simulink model "ROS_DJI_waypoint_follower"  (R2020b)
settings: Solver=FixedStepDiscrete  StartTime=0.0  StopTime=inf  FixedStep=0.001  RelTol=1e-3  EnableMultiTasking=on
model workspace (MAT data in the model file):
  SL_ROS_VariableLengthArrays_MaxSizes.CommonInfo.ArrayTruncateAction = 'EmitWarning'
  SL_ROS_VariableLengthArrays_MaxSizes.MsgTypeMap = containers.Map
  SL_ROS_VariableLengthArrays_MaxSizes.MsgTypeMap.serialization.keys = {'geometry_msgs/PoseArray', 'sensor_msgs/Joy'}
  SL_ROS_VariableLengthArrays_MaxSizes.MsgTypeMap.serialization.values{1}.PropertyName = 'Poses'
  SL_ROS_VariableLengthArrays_MaxSizes.MsgTypeMap.serialization.values{1}.DataType = 'geometry_msgs/Pose'
  SL_ROS_VariableLengthArrays_MaxSizes.MsgTypeMap.serialization.values{1}.MaxLength = 255
  SL_ROS_VariableLengthArrays_MaxSizes.MsgTypeMap.serialization.values{2}(1).PropertyName = 'Axes'
  SL_ROS_VariableLengthArrays_MaxSizes.MsgTypeMap.serialization.values{2}(1).DataType = 'single'
  SL_ROS_VariableLengthArrays_MaxSizes.MsgTypeMap.serialization.values{2}(1).MaxLength = 4
  SL_ROS_VariableLengthArrays_MaxSizes.MsgTypeMap.serialization.values{2}(2).PropertyName = 'Buttons'
  SL_ROS_VariableLengthArrays_MaxSizes.MsgTypeMap.serialization.values{2}(2).DataType = 'int32'
  SL_ROS_VariableLengthArrays_MaxSizes.MsgTypeMap.serialization.values{2}(2).MaxLength = 128
  SL_ROS_VariableLengthArrays_MaxSizes.MsgTypeMap.serialization.uniformity = 0
  SL_ROS_VariableLengthArrays_MaxSizes.MsgTypeMap.serialization.keyType = 'char'
  SL_ROS_VariableLengthArrays_MaxSizes.MsgTypeMap.serialization.valueType = 'any'
undefined symbols (not defined in the file or in its folder): DJIServiceDroneTaskControl
libraries: robotlib x13, simulink x5, uavutilslib x1, uavalgslib x1
settings Model: EnablePacing=on  Creator=The MathWorks, Inc.  LastModifiedBy=kritika
settings DataIOCC: LimitDataPoints=on  SaveFormat=Array  ReturnWorkspaceOutputs=off
settings OptimizationCC: ZeroExternalMemoryAtStartup=off  ZeroInternalMemoryAtStartup=off  LifeSpan=1  MaxStackSize=64  EfficientTunableParamExpr=on
settings DebuggingCC: SolverPrmCheckMsg=warning  SFUnexpectedBacktrackingDiag=warning  SFNoUnconditionalDefaultTransitionDiag=warning  SFExecutionAtInitializationDiag=none  ArithmeticOperatorsInVariantConditions=warning
settings HardwareCC: ProdBitPerPointer=32  ProdBitPerSizeT=32  ProdBitPerPtrDiffT=32  ProdLargestAtomicFloat=None  ProdIntDivRoundTo=Undefined  ProdEndianess=Unspecified  ProdWordSize=32  ProdHWDeviceType=Generic->Unspecified (assume 32-bit Generic)  TargetHWDeviceType=Generic->Unspecified (assume 32-bit Generic)
settings ModelReferenceCC: PropagateSignalLabelsOutOfModel=off
settings SFSimCC: SimUseLocalCustomCode=off  CustomCodeUndefinedFunction=UseInterfaceOnly  SimTargetLang=C++
settings RTWCC: Description=Embedded Coder  SystemTargetFile=ert.tlc  HardwareBoard=Robot Operating System (ROS)  TLCOptions=-aInlineSetEventsForThisBaseRateFcn=TLC_FALSE -aSuppressMultiTaskScheduler=TLC_FALSE -aRateBasedStepFcn=0  TemplateMakefile=ert_default_tmf  RTWUseLocalCustomCode=off  Toolchain=Catkin  TargetLang=C++
settings CodeAppCC: StateflowObjectComments=on
settings ERTTargetCC: MultiwordLength=2048  ERTCustomFileBanners=off  CodeInterfacePackaging=C++ class  SupportContinuousTime=on  SupportNonInlinedSFcns=on  RemoveResetFunc=off  SupportVariableSizeSignals=on  ModelStepFunctionPrototypeControlCompliant=off  RootIOFormat=Structure reference  ConvertIfToSwitch=off  SuppressUnreachableDefaultCases=off
settings ConfigComp: CovMetricSettings=dw  CovSaveCumulativeToWorkspaceVar=on  CovSaveSingleToWorkspaceVar=on  CovExternalEMLEnable=off  CovSFcnEnable=off

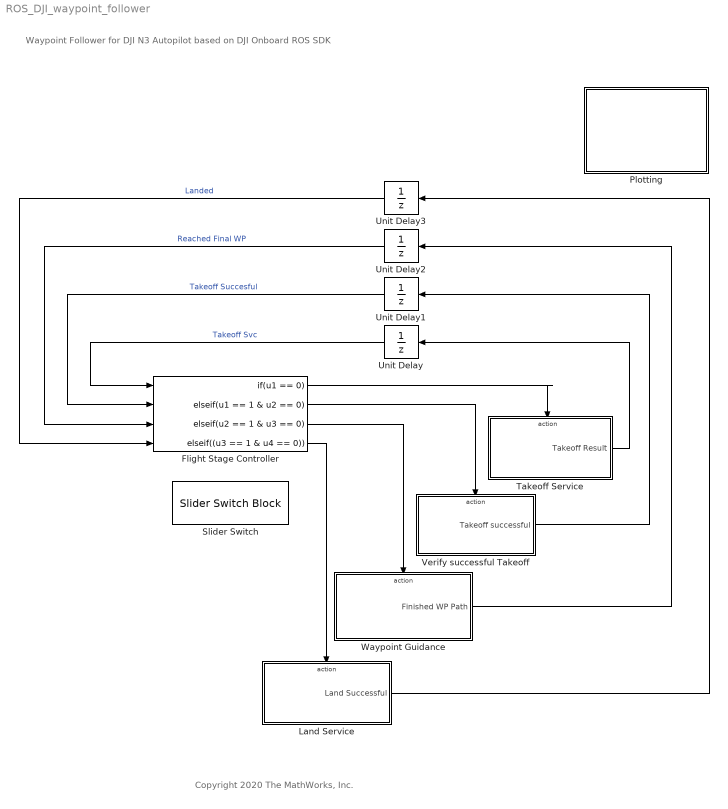
== system ROS_DJI_waypoint_follower ==
  note: Copyright 2020 The MathWorks, Inc.
  note: Waypoint Follower for DJI N3 Autopilot based on DJI Onboard ROS SDK
  Flight Stage Controller : If  NumInputs=4  IfExpression=u1 == 0  ElseIfExpressions=u1 == 1 & u2 == 0, u2 == 1 & u3 == 0, (u3 == 1 & u4 == 0)  ShowElse=off
  Land Service : Subsystem  TreatAsAtomicUnit=on
  Plotting : Subsystem
  Slider Switch : SliderSwitchBlock
      settings: Values={{'Off', 'On'}, [0 1]}
  Takeoff Service : Subsystem
  Unit Delay{,1..3} (4 alike) : UnitDelay  SampleTime=-1  HasFrameUpgradeWarning=on
  Verify successful Takeoff : Subsystem
  Waypoint Guidance : Subsystem
  wires:
  Unit Delay/1 -> Flight Stage Controller/1  "Takeoff Svc"
  Flight Stage Controller/1 -> Takeoff Service/Action
  Takeoff Service/1(Takeoff Result) -> Unit Delay/1
  Flight Stage Controller/2 -> Verify successful Takeoff/Action
  Verify successful Takeoff/1(Takeoff successful) -> Unit Delay1/1
  Unit Delay1/1 -> Flight Stage Controller/2  "Takeoff Succesful"
  Flight Stage Controller/3 -> Waypoint Guidance/Action
  Waypoint Guidance/1(Finished WP Path) -> Unit Delay2/1
  Unit Delay2/1 -> Flight Stage Controller/3  "Reached Final WP"
  Flight Stage Controller/4 -> Land Service/Action
  Land Service/1(Land Successful) -> Unit Delay3/1
  Unit Delay3/1 -> Flight Stage Controller/4  "Landed"

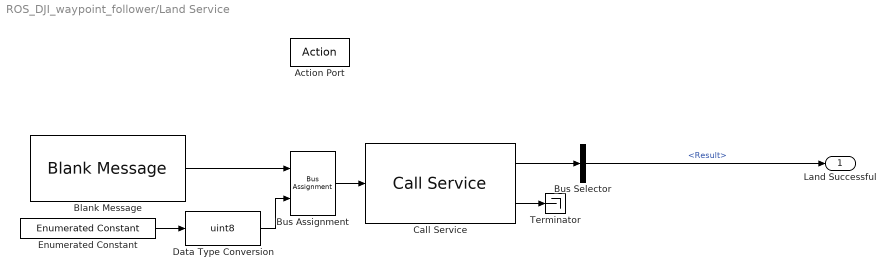
== system ROS_DJI_waypoint_follower/Land Service ==
  Action Port : ActionPort  ActionPortLabel=elseif( (u3 == 1 & u4 == 0))
  Blank Message : robotlib/Blank Message  messageClass=Service Request  entityType=std_srvs/Empty  messageType=std_srvs/EmptyRequest  SampleTime=-1  legacyBusStruct=off
  Bus Assignment : BusAssignment  AssignedSignals=Task
  Bus Selector : BusSelector  OutputSignals=Result
  Call Service : robotlib/Call Service  topicSource=Select from ROS network  service=/dji_sdk/drone_task_control  serviceType=dji_sdk/DroneTaskControl  connectionTimeout=5  keepPersistent=off  ShowErrorCodeOutput=on  legacyBusStruct=off
      settings: SourceProductBaseCode=RR
  Data Type Conversion : DataTypeConversion  OutDataTypeStr=uint8
  Enumerated Constant : simulink/Sources/Enumerated Constant  OutDataTypeStr=Enum: DJIServiceDroneTaskControl  Value=DJIServiceDroneTaskControl.Landing  SampleTime=Inf
  Terminator : Terminator
  Land Successful : Outport
  wires:
  Blank Message/1 -> Bus Assignment/1
  Bus Assignment/1 -> Call Service/1
  Enumerated Constant/1 -> Data Type Conversion/1
  Data Type Conversion/1 -> Bus Assignment/2
  Call Service/2 -> Terminator/1
  Call Service/1 -> Bus Selector/1
  Bus Selector/1 -> Land Successful/1  "<Result>"

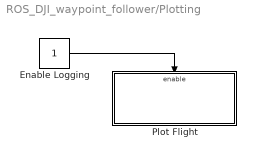
== system ROS_DJI_waypoint_follower/Plotting ==
  Enable Logging : Constant
  Plot Flight : Subsystem
  wires:
  Enable Logging/1 -> Plot Flight/Enable

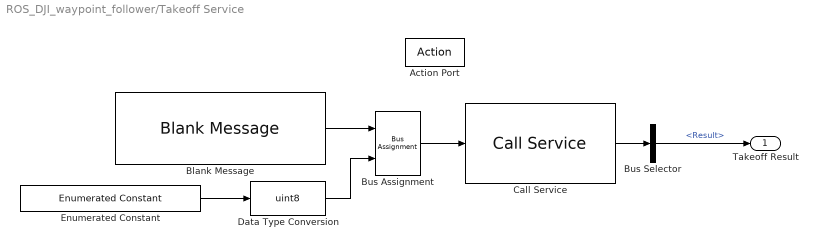
== system ROS_DJI_waypoint_follower/Takeoff Service ==
  Action Port : ActionPort  ActionPortLabel=if(u1 == 0)
  Blank Message : robotlib/Blank Message  messageClass=Service Request  entityType=std_srvs/Empty  messageType=std_srvs/EmptyRequest  SampleTime=-1  legacyBusStruct=off
  Bus Assignment : BusAssignment  AssignedSignals=Task
  Bus Selector : BusSelector  OutputSignals=Result
  Call Service : robotlib/Call Service  topicSource=Select from ROS network  service=/dji_sdk/drone_task_control  serviceType=dji_sdk/DroneTaskControl  connectionTimeout=5  keepPersistent=off  ShowErrorCodeOutput=off  legacyBusStruct=off
      settings: SourceProductBaseCode=RR
  Data Type Conversion : DataTypeConversion  OutDataTypeStr=uint8
  Enumerated Constant : simulink/Sources/Enumerated Constant  OutDataTypeStr=Enum: DJIServiceDroneTaskControl  Value=DJIServiceDroneTaskControl.TakeOff  SampleTime=Inf
  Takeoff Result : Outport
  wires:
  Data Type Conversion/1 -> Bus Assignment/2
  Call Service/1 -> Bus Selector/1
  Blank Message/1 -> Bus Assignment/1
  Enumerated Constant/1 -> Data Type Conversion/1
  Bus Selector/1 -> Takeoff Result/1  "<Result>"
  Bus Assignment/1 -> Call Service/1

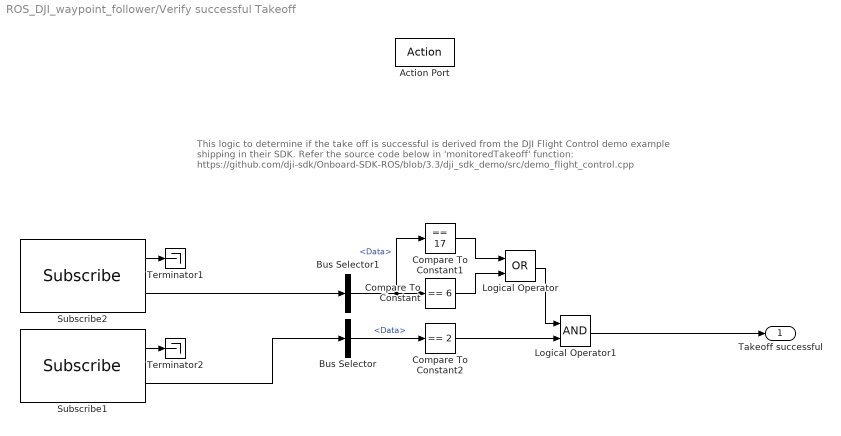
== system ROS_DJI_waypoint_follower/Verify successful Takeoff ==
  note: This logic to determine if the take off is successful is derived from the DJI Flight Control demo example
      | shipping in their SDK.
      |
      | Refer the source code below in 'monitoredTakeoff' function:
      | https://github.com/dji-sdk/Onboard-SDK-ROS/blob/3.3/dji_sdk_demo/src/demo_flight_control.cpp
  Action Port : ActionPort  ActionPortLabel=elseif(u1 == 1 & u2 == 0)
  Bus Selector : BusSelector  OutputSignals=Data
  Bus Selector1 : BusSelector  OutputSignals=Data
  Compare To Constant : simulink/Logic and Bit Operations/Compare To Constant  relop===  const=6  OutDataTypeStr=boolean
  Compare To Constant1 : simulink/Logic and Bit Operations/Compare To Constant  relop===  const=17  OutDataTypeStr=boolean
  Compare To Constant2 : simulink/Logic and Bit Operations/Compare To Constant  relop===  const=2  OutDataTypeStr=boolean
  Logical Operator : Logic  Operator=OR  AllPortsSameDT=off  OutDataTypeStr=boolean
  Logical Operator1 : Logic  AllPortsSameDT=off  OutDataTypeStr=boolean
  Subscribe1 : robotlib/Subscribe  topicSource=Select from ROS network  topic=/dji_sdk/flight_status  messageType=std_msgs/UInt8  SampleTime=-1  legacyBusStruct=off  messageQueueLength=51
  Subscribe2 : robotlib/Subscribe  topicSource=Select from ROS network  topic=/dji_sdk/display_mode  messageType=std_msgs/UInt8  SampleTime=-1  legacyBusStruct=off  messageQueueLength=51
  Terminator1 : Terminator
  Terminator2 : Terminator
  Takeoff successful : Outport
  wires:
  Logical Operator1/1 -> Takeoff successful/1
  Subscribe1/1 -> Terminator2/1
  Subscribe2/1 -> Terminator1/1
  Subscribe2/2 -> Bus Selector1/1
  Subscribe1/2 -> Bus Selector/1
  Bus Selector1/1 -> Compare To Constant1/1, Compare To Constant/1  "<Data>"
  Bus Selector/1 -> Compare To Constant2/1  "<Data>"
  Compare To Constant1/1 -> Logical Operator/1
  Compare To Constant/1 -> Logical Operator/2
  Compare To Constant2/1 -> Logical Operator1/2
  Logical Operator/1 -> Logical Operator1/1

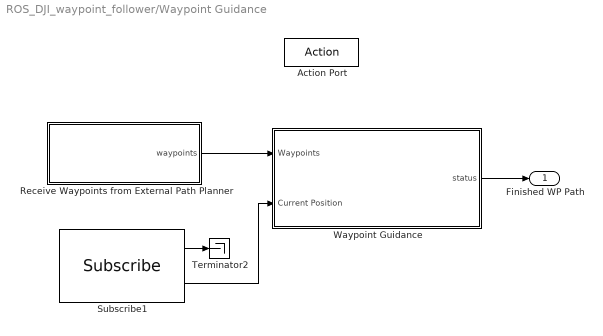
== system ROS_DJI_waypoint_follower/Waypoint Guidance ==
  Action Port : ActionPort  PropagateVarSize=During execution  ActionPortLabel=elseif( u2 == 1 & u3 == 0)
  Receive Waypoints from External Path Planner : Subsystem
  Subscribe1 : robotlib/Subscribe  topicSource=Select from ROS network  topic=/dji_sdk/local_position  messageType=geometry_msgs/PointStamped  SampleTime=-1  legacyBusStruct=off  messageQueueLength=51
  Terminator2 : Terminator
  Waypoint Guidance : Subsystem
  Finished WP Path : Outport
  wires:
  Subscribe1/2 -> Waypoint Guidance/2(Current Position)
  Receive Waypoints from External Path Planner/1(waypoints) -> Waypoint Guidance/1(Waypoints)
  Waypoint Guidance/1("status ") -> Finished WP Path/1
  Subscribe1/1 -> Terminator2/1

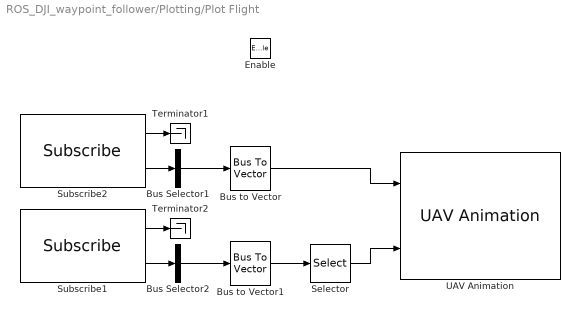
== system ROS_DJI_waypoint_follower/Plotting/Plot Flight ==
  Enable : EnablePort
  Bus Selector1 : BusSelector  DialogController=Simulink.DDGSource_BusSelector  OutputSignals=Point  OutputAsBus=on
  Bus Selector2 : BusSelector  DialogController=Simulink.DDGSource_BusSelector  OutputSignals=Quaternion  OutputAsBus=on
  Bus to Vector : BusToVector
  Bus to Vector1 : BusToVector
  Selector : Selector  InputPortWidth=4  IndexOptions=Index vector (dialog)  Indices=[4 1 2 3]  OutputSizes=1
  Subscribe1 : robotlib/Subscribe  topicSource=Select from ROS network  topic=/dji_sdk/attitude  messageType=geometry_msgs/QuaternionStamped  SampleTime=-1  legacyBusStruct=off  messageQueueLength=51
  Subscribe2 : robotlib/Subscribe  topicSource=Specify your own  topic=/dji_sdk/local_position  messageType=geometry_msgs/PointStamped  SampleTime=-1  legacyBusStruct=off  messageQueueLength=51
  Terminator1 : Terminator
  Terminator2 : Terminator
  UAV Animation : uavutilslib/UAV Animation  UAVType=Multirotor  UAVSize=10  InertialZDirection=Up  SampleTime=-1
      settings: SourceProductBaseCode=UV
  wires:
  Subscribe2/1 -> Terminator1/1
  Subscribe2/2 -> Bus Selector1/1
  Bus Selector1/1 -> Bus to Vector/1
  Bus to Vector1/1 -> Selector/1
  Subscribe1/1 -> Terminator2/1
  Bus Selector2/1 -> Bus to Vector1/1
  Subscribe1/2 -> Bus Selector2/1
  Bus to Vector/1 -> UAV Animation/1
  Selector/1 -> UAV Animation/2

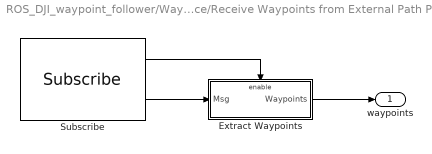
== system ROS_DJI_waypoint_follower/Waypoint Guidance/Receive Waypoints from External Path Planner ==
  Extract Waypoints : Subsystem
  Subscribe : robotlib/Subscribe  topicSource=Specify your own  topic=/waypoints  messageType=geometry_msgs/PoseArray  SampleTime=-1  legacyBusStruct=off  messageQueueLength=1
  waypoints : Outport
  wires:
  Extract Waypoints/1(Waypoints) -> waypoints/1
  Subscribe/2 -> Extract Waypoints/1(Msg)
  Subscribe/1 -> Extract Waypoints/Enable

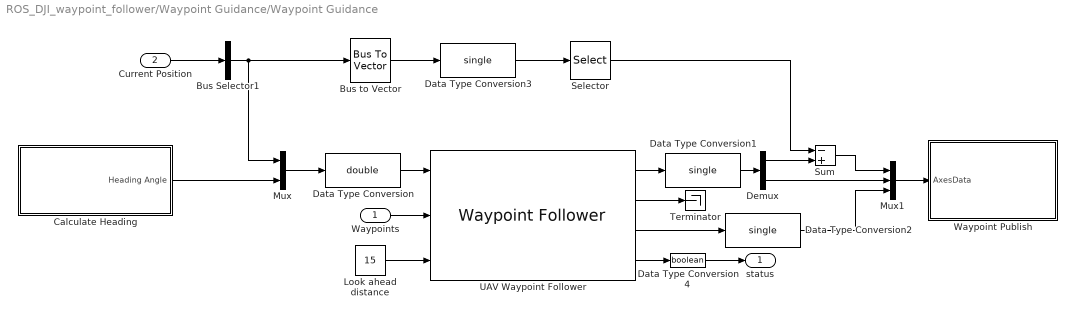
== system ROS_DJI_waypoint_follower/Waypoint Guidance/Waypoint Guidance ==
  Waypoints : Inport
  Current Position : Inport  Port=2
  Bus Selector1 : BusSelector  DialogController=Simulink.DDGSource_BusSelector  OutputSignals=Point  OutputAsBus=on
  Bus to Vector : BusToVector
  Calculate Heading : Subsystem
  Data Type Conversion : DataTypeConversion  OutDataTypeStr=double
  Data Type Conversion1 : DataTypeConversion  OutDataTypeStr=single
  Data Type Conversion2 : DataTypeConversion  OutDataTypeStr=single
  Data Type Conversion3 : DataTypeConversion  OutDataTypeStr=single
  Data Type Conversion4 : DataTypeConversion  OutDataTypeStr=boolean
  Demux : Demux  Outputs=[2 1]
  Look ahead distance : Constant  Value=15  SampleTime=-1
  Mux : Mux  Inputs=2
  Mux1 : Mux  Inputs=3
  Selector : Selector  InputPortWidth=3  IndexOptions=Index vector (dialog)  Indices=[1 2]  OutputSizes=1
  Sum : Sum  Inputs=-+
  Terminator : Terminator
  UAV Waypoint Follower : uavalgslib/Waypoint Follower  UAVType=multirotor  StartFrom=first  TransitionRadiusSource=internal  TransitionRadius=10  YawInput=off  ShowCrossTrackErrorOutput=off  ShowStatusOutput=on  SimulateUsing=Interpreted execution
      settings: SourceProductBaseCode=UV
  Waypoint Publish : Subsystem  TreatAsAtomicUnit=on
  "status " : Outport
  wires:
  Demux/2 -> Mux1/2
  Data Type Conversion1/1 -> Demux/1
  UAV Waypoint Follower/4 -> Data Type Conversion4/1
  Data Type Conversion2/1 -> Mux1/3
  Sum/1 -> Mux1/1
  Data Type Conversion3/1 -> Selector/1
  Bus to Vector/1 -> Data Type Conversion3/1
  Calculate Heading/1(Heading Angle) -> Mux/2
  Bus Selector1/1 -> Bus to Vector/1, Mux/1
  Data Type Conversion/1 -> UAV Waypoint Follower/1
  UAV Waypoint Follower/1 -> Data Type Conversion1/1
  UAV Waypoint Follower/2 -> Terminator/1
  Look ahead distance/1 -> UAV Waypoint Follower/3
  UAV Waypoint Follower/3 -> Data Type Conversion2/1
  Waypoints/1 -> UAV Waypoint Follower/2
  Mux1/1 -> Waypoint Publish/1(AxesData)
  Current Position/1 -> Bus Selector1/1
  Mux/1 -> Data Type Conversion/1
  Selector/1 -> Sum/1
  Demux/1 -> Sum/2
  Data Type Conversion4/1 -> "status "/1

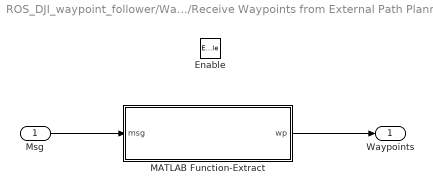
== system ROS_DJI_waypoint_follower/Waypoint Guidance/Receive Waypoints from External Path Planner/Extract Waypoints ==
  Msg : Inport
  Enable : EnablePort  PropagateVarSize=During execution
  MATLAB Function-Extract : MATLAB Function  TreatAsAtomicUnit=on
  Waypoints : Outport
  wires:
  MATLAB Function-Extract/1(wp) -> Waypoints/1
  Msg/1 -> MATLAB Function-Extract/1(msg)

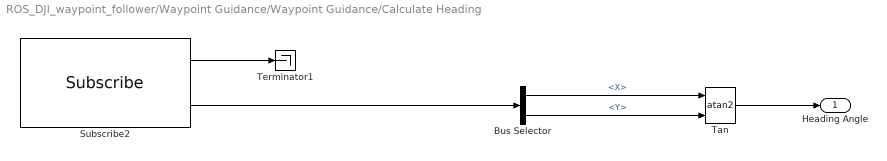
== system ROS_DJI_waypoint_follower/Waypoint Guidance/Waypoint Guidance/Calculate Heading ==
  Bus Selector : BusSelector  OutputSignals=Vector_.X,Vector_.Y
  Subscribe2 : robotlib/Subscribe  topicSource=Select from ROS network  topic=/dji_sdk/velocity  messageType=geometry_msgs/Vector3Stamped  SampleTime=-1  legacyBusStruct=off  messageQueueLength=51
  Tan : Trigonometry  Operator=atan2
  Terminator1 : Terminator
  Heading Angle : Outport
  wires:
  Subscribe2/2 -> Bus Selector/1
  Bus Selector/2 -> Tan/2  "<Y>"
  Bus Selector/1 -> Tan/1  "<X>"
  Subscribe2/1 -> Terminator1/1
  Tan/1 -> Heading Angle/1

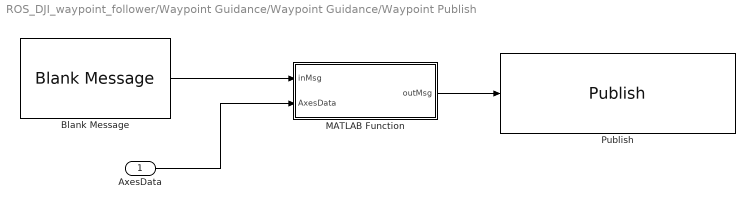
== system ROS_DJI_waypoint_follower/Waypoint Guidance/Waypoint Guidance/Waypoint Publish ==
  AxesData : Inport
  Blank Message : robotlib/Blank Message  messageClass=Message  entityType=sensor_msgs/Joy  messageType=sensor_msgs/Joy  SampleTime=-1  legacyBusStruct=off
  MATLAB Function : MATLAB Function  TreatAsAtomicUnit=on
  Publish : robotlib/Publish  topicSource=Specify your own  topic=/dji_sdk/flight_control_setpoint_ENUposition_yaw  messageType=sensor_msgs/Joy  legacyBusStruct=off  messageQueueLength=1
  wires:
  AxesData/1 -> MATLAB Function/2(AxesData)
  Blank Message/1 -> MATLAB Function/1(inMsg)
  MATLAB Function/1(outMsg) -> Publish/1

== matlab function ROS_DJI_waypoint_follower/Waypoint Guidance/Receive Waypoints from External Path Planner/Extract Waypoints/MATLAB Function-Extract ==
  data: msg input; wp output size=[255 3]
function wp  = extractNestedArrayMessages(msg)
%#codegen

% geometry_msgs/PoseArray consists of
%          Header: [1x1 Header]
%           Poses: [nx1 Pose]

% Poses is an array of "geometry_msgs/Pose", which consists of
%        Position: [1x1 Point]
%     Orientation: [1x1 Quaternion]

% Position is "geometry_msgs/Point", which consists of
%               X: 0
%               Y: 0
%               Z: 0

% Orientation is "geometry_msgs/Quaternion", which consists of
%               X: 0
%               Y: 0
%               Z: 0
%               W: 0

% Extract elements from an array with specified indices (1,2) and extract
% information from those elements

X = zeros(numel(msg.Poses),1);
Y = zeros(numel(msg.Poses),1);
Z = zeros(numel(msg.Poses),1);
for i=1:numel(msg.Poses)
    X(i) = msg.Poses(i).Position.X;
    Y(i) = msg.Poses(i).Position.Y;
    Z(i) = msg.Poses(i).Position.Z;
end
wp = [X Y Z];

lv = [false(1,3); wp(1:end-1,:) == wp(2:end,:)];
s = sum(lv,2);
del_r = find(s==3);
wp(del_r,:)=[];

== matlab function ROS_DJI_waypoint_follower/Waypoint Guidance/Waypoint Guidance/Waypoint Publish/MATLAB Function ==
  data: inMsg input Bus: SL_Bus_ROS_DJI_waypoint_follower_sensor_msgs_Joy; outMsg output Bus: SL_Bus_ROS_DJI_waypoint_follower_sensor_msgs_Joy; AxesData input single
function outMsg = fcn(inMsg, AxesData)

inMsg.Axes = AxesData;
inMsg.Axes_SL_Info.CurrentLength = uint32(numel(AxesData));
inMsg.Axes_SL_Info.ReceivedLength = uint32(numel(AxesData));

outMsg = inMsg;
